simulink model "mcu"  (R2025b)
settings: Solver=FixedStepDiscrete  StartTime=0.0  StopTime=10.0  FixedStep=Ts_inner  RelTol=1e-3
undefined symbols (not defined in the file): controller, imu, mahony, quadcop, safety, Ts_batt, Ts_inner
settings Model: DataDictionary=project.sldd  Creator=Nick  LastModifiedBy=Rakete
settings SolverCC: AutoInsertRateTranBlk=on
settings OptimizationCC: DefaultParameterBehavior=Inlined  EnhancedBackFolding=on  PassReuseOutputArgsAs=Individual arguments  ZeroExternalMemoryAtStartup=off  ZeroInternalMemoryAtStartup=off  OptimizeBlockOrder=speed  DifferentSizesBufferReuse=on  OptimizationCustomize=off  EfficientTunableParamExpr=on
settings DebuggingCC: ParameterTunabilityLossMsg=error
settings HardwareCC: ProdBitPerPointer=32.0  ProdBitPerSizeT=32.0  ProdBitPerPtrDiffT=32.0  ProdLargestAtomicInteger=Long  ProdLargestAtomicFloat=Double  ProdWordSize=32.0  ProdLongLongMode=on  ProdHWDeviceType=ARM Compatible->ARM Cortex-M
settings SFSimCC: MATLABDynamicMemAlloc=off
settings RTWCC: SystemTargetFile=ert.tlc  GenCodeOnly=on  PackageGeneratedCodeAndArtifacts=on  TemplateMakefile=ert_default_tmf  GenerateReport=on  TargetLang=C++  Description=Embedded Coder
settings CodeAppCC: ForceParamTrailComments=on  IgnoreCustomStorageClasses=off  OperatorAnnotations=on  SimulinkDataObjDesc=on  SFDataObjDesc=on  InsertBlockDesc=on
settings ERTTargetCC: RootIOFormat=Structure reference  ERTCustomFileTemplate=example_file_process.tlc  TargetLangStandard=C++11 (ISO)  GenerateSampleERTMain=on  CodeInterfacePackaging=C++ class  SubcomponentCodeInterfacePackaging=C++ class  SupportNonFinite=off

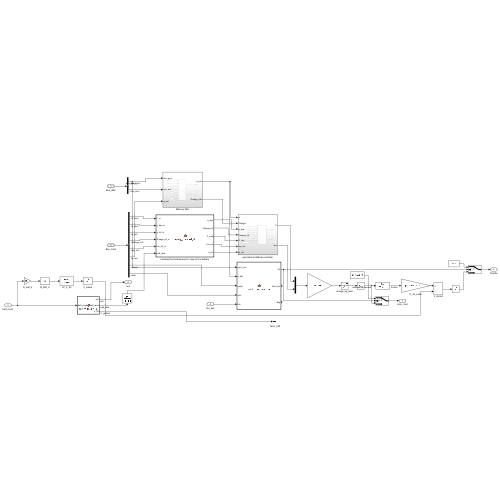
[thumbnail: Simulink's stored preview of the top-level diagram]
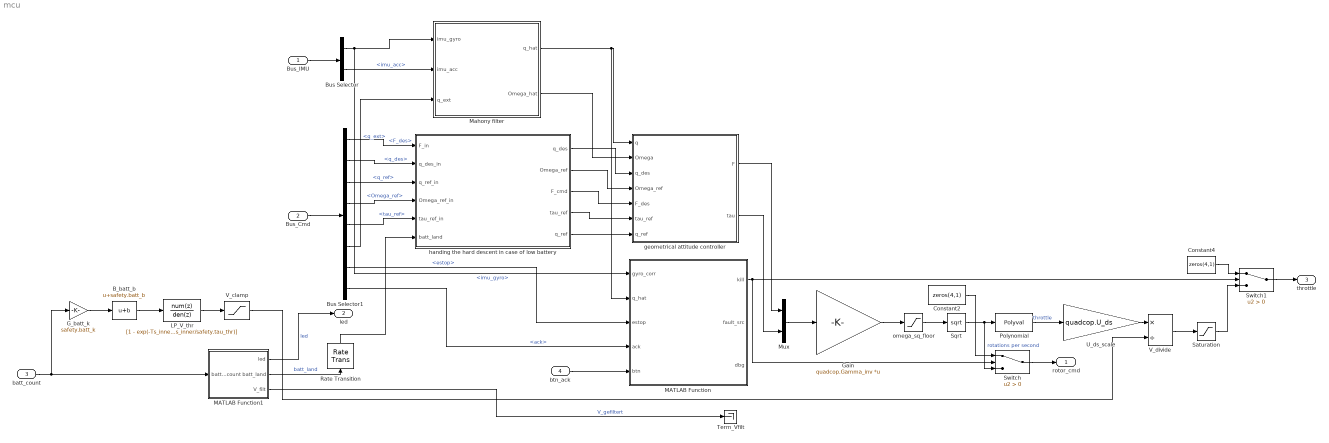
== system mcu ==
  Bus_IMU : Inport  OutDataTypeStr=Bus: Bus_IMU
  Bus_Cmd : Inport  Port=2  OutDataTypeStr=Bus: Bus_Cmd
  batt_count : Inport  Port=3
  btn_ack : Inport  Port=4  OutDataTypeStr=boolean
  B_batt_b : Bias  Bias=safety.batt_b  SaturateOnIntegerOverflow=off
  Bus Selector : BusSelector  OutputSignals=imu_gyro,imu_acc
  Bus Selector1 : BusSelector  OutputSignals=F_des,q_des,q_ref,Omega_ref,tau_ref,q_ext,estop,ack
  Constant2 : Constant  Value=zeros(4,1)
  Constant4 : Constant  Value=zeros(4,1)
  G_batt_k : Gain  Gain=safety.batt_k
  Gain : Gain  Gain=quadcop.Gamma_inv  Multiplication=Matrix(K*u) (u vector)
  LP_V_thr : DiscreteTransferFcn  Numerator=[1 - exp(-Ts_inner/safety.tau_thr)]  Denominator=[1, -exp(-Ts_inner/safety.tau_thr)]  InitialStates=quadcop.V_thr_init  SampleTime=Ts_inner
  MATLAB Function : MATLAB Function  TreatAsAtomicUnit=on
  MATLAB Function1 : MATLAB Function  TreatAsAtomicUnit=on  SystemSampleTime=Ts_batt
  Mahony filter : Subsystem
  Mux : Mux  Inputs=2
  Polynomial : Polyval  Coefs=quadcop.p_from_omega
  Rate Transition : RateTransition  OutPortSampleTime=Ts_inner
  Saturation : Saturate  UpperLimit=100  LowerLimit=0
  Sqrt : Sqrt
  Switch : Switch  Criteria=u2 > Threshold  SaturateOnIntegerOverflow=off  InputSameDT=off
  Switch1 : Switch  Criteria=u2 > Threshold  SaturateOnIntegerOverflow=off  InputSameDT=off
  Term_Vfilt : Terminator
  U_ds_scale : Gain  Gain=quadcop.U_ds
  V_clamp : Saturate  UpperLimit=quadcop.V_thr_max  LowerLimit=quadcop.V_thr_min
  V_divide : Product  Inputs=*/
  geometrical attitude controller : Subsystem
  handing the hard descent in case of low battery : MATLAB Function  TreatAsAtomicUnit=on  SystemSampleTime=Ts_inner
  omega_sq_floor : Saturate  UpperLimit=inf  LowerLimit=0
  rotor_cmd : Outport
  led : Outport  Port=2
  throttle : Outport  Port=3
  wires:
  Bus_IMU/1 -> Bus Selector/1
  geometrical attitude controller/2(tau) -> Mux/2
  Bus Selector/2 -> Mahony filter/2(imu_acc)  "<imu_acc>"
  Bus_Cmd/1 -> Bus Selector1/1
  Bus Selector/1 -> MATLAB Function/1(gyro_corr), Mahony filter/1(imu_gyro)  "<imu_gyro>"
  Bus Selector1/1 -> handing the hard descent in case of low battery/1(F_in)  "<F_des>"
  Bus Selector1/2 -> handing the hard descent in case of low battery/2(q_des_in)  "<q_des>"
  Bus Selector1/3 -> handing the hard descent in case of low battery/3(q_ref_in)  "<q_ref>"
  Bus Selector1/4 -> handing the hard descent in case of low battery/4(Omega_ref_in)  "<Omega_ref>"
  Mux/1 -> Gain/1
  Mahony filter/1(q_hat) -> geometrical attitude controller/1(q), MATLAB Function/2(q_hat)
  Bus Selector1/5 -> handing the hard descent in case of low battery/5(tau_ref_in)  "<tau_ref>"
  handing the hard descent in case of low battery/4(tau_ref) -> geometrical attitude controller/6(tau_ref)
  Bus Selector1/6 -> Mahony filter/3(q_ext)  "<q_ext>"
  Bus Selector1/7 -> MATLAB Function/3(estop)  "<estop>"
  Bus Selector1/8 -> MATLAB Function/4(ack)  "<ack>"
  Rate Transition/1 -> handing the hard descent in case of low battery/6(batt_land)
  Mahony filter/2(Omega_hat) -> geometrical attitude controller/2(Omega)
  Saturation/1 -> Switch1/3
  handing the hard descent in case of low battery/1(q_des) -> geometrical attitude controller/3(q_des)
  handing the hard descent in case of low battery/2(Omega_ref) -> geometrical attitude controller/4(Omega_ref)
  Constant2/1 -> Switch/1
  handing the hard descent in case of low battery/3(F_cmd) -> geometrical attitude controller/5(F_des)
  handing the hard descent in case of low battery/5(q_ref) -> geometrical attitude controller/7(q_ref)
  btn_ack/1 -> MATLAB Function/5(btn)
  geometrical attitude controller/1(F) -> Mux/1
  MATLAB Function/1(kill) -> Switch/2, Switch1/2
  V_divide/1 -> Saturation/1
  Sqrt/1 -> Switch/3, Polynomial/1  "rotations per second"
  Polynomial/1 -> U_ds_scale/1  "throttle"
  Switch/1 -> rotor_cmd/1
  U_ds_scale/1 -> V_divide/1
  Constant4/1 -> Switch1/1
  Switch1/1 -> throttle/1
  Gain/1 -> omega_sq_floor/1
  omega_sq_floor/1 -> Sqrt/1
  MATLAB Function1/3(V_filt) -> Term_Vfilt/1  "V_gefiltert"
  LP_V_thr/1 -> V_clamp/1
  B_batt_b/1 -> LP_V_thr/1
  G_batt_k/1 -> B_batt_b/1
  V_clamp/1 -> V_divide/2
  MATLAB Function1/2(batt_land) -> Rate Transition/1  "batt_land"
  MATLAB Function1/1(led) -> led/1  "led"
  batt_count/1 -> G_batt_k/1, MATLAB Function1/1(batt_count)

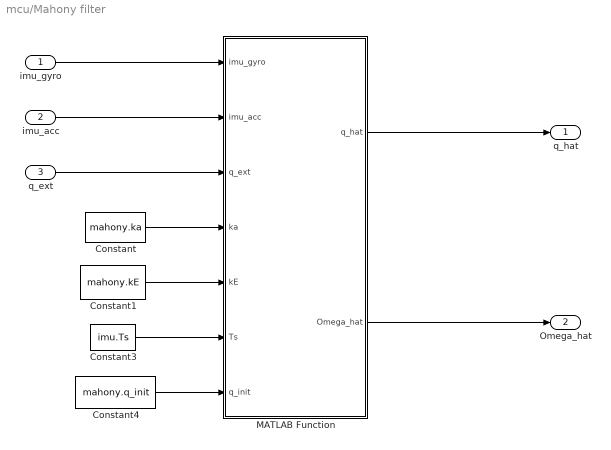
== system mcu/Mahony filter ==
  imu_gyro : Inport
  imu_acc : Inport  Port=2
  q_ext : Inport  Port=3
  Constant : Constant  Value=mahony.ka
  Constant1 : Constant  Value=mahony.kE
  Constant3 : Constant  Value=imu.Ts
  Constant4 : Constant  Value=mahony.q_init
  MATLAB Function : MATLAB Function  TreatAsAtomicUnit=on
  q_hat : Outport
  Omega_hat : Outport  Port=2
  wires:
  MATLAB Function/1(q_hat) -> q_hat/1
  MATLAB Function/2(Omega_hat) -> Omega_hat/1
  imu_gyro/1 -> MATLAB Function/1(imu_gyro)
  imu_acc/1 -> MATLAB Function/2(imu_acc)
  q_ext/1 -> MATLAB Function/3(q_ext)
  Constant/1 -> MATLAB Function/4(ka)
  Constant1/1 -> MATLAB Function/5(kE)
  Constant3/1 -> MATLAB Function/6(Ts)
  Constant4/1 -> MATLAB Function/7(q_init)

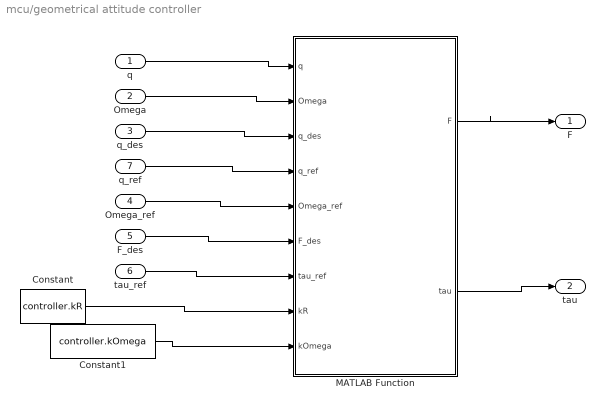
== system mcu/geometrical attitude controller ==
  q : Inport
  Omega : Inport  Port=2
  q_des : Inport  Port=3
  Omega_ref : Inport  Port=4
  F_des : Inport  Port=5
  tau_ref : Inport  Port=6
  q_ref : Inport  Port=7
  Constant : Constant  Value=controller.kR
  Constant1 : Constant  Value=controller.kOmega
  MATLAB Function : MATLAB Function  TreatAsAtomicUnit=on
  F : Outport
  tau : Outport  Port=2
  wires:
  MATLAB Function/1(F) -> F/1
  MATLAB Function/2(tau) -> tau/1
  q/1 -> MATLAB Function/1(q)
  Omega/1 -> MATLAB Function/2(Omega)
  q_des/1 -> MATLAB Function/3(q_des)
  Omega_ref/1 -> MATLAB Function/5(Omega_ref)
  F_des/1 -> MATLAB Function/6(F_des)
  tau_ref/1 -> MATLAB Function/7(tau_ref)
  Constant/1 -> MATLAB Function/8(kR)
  Constant1/1 -> MATLAB Function/9(kOmega)
  q_ref/1 -> MATLAB Function/4(q_ref)

== matlab function mcu/geometrical attitude controller/MATLAB Function ==
  data: q input; F output; Omega input; q_des input; q_ref input; Omega_ref input; F_des input; tau_ref input; kR input; kOmega input; tau output; quadcop parameter
function [F, tau] = geo_attitude_ctrl_sl(q, Omega, q_des, q_ref, Omega_ref, F_des, tau_ref, kR, kOmega, quadcop)
%#codegen
% WRAPPER — code liegt in
% scripts\functions\geo_attitude_ctrl.m - dieser Block ruft sie nur auf
[F, tau] = geo_attitude_ctrl(q, Omega, q_des, q_ref, Omega_ref, F_des, tau_ref, kR, kOmega, quadcop.J);
end

== matlab function mcu/Mahony filter/MATLAB Function ==
  data: imu_gyro input; q_hat output; imu_acc input; q_ext input; ka input; kE input; Ts input; Omega_hat output; q_init input
function [q_hat, Omega_hat] = mahony_filter_sl(imu_gyro, imu_acc, q_ext, ka, kE, Ts, q_init)
%#codegen
% WRAPPER — code liegt in
% scripts\functions\mahony_filter.m - dieser Block ruft sie nur auf
[q_hat, Omega_hat] = mahony_filter(imu_gyro, imu_acc, q_ext, ka, kE, Ts, q_init);
end

== matlab function mcu/MATLAB Function ==
  data: gyro_corr input double size=[3 1]; q_hat input; estop input uint8 size=1; kill output boolean size=1; ack input boolean size=1; btn input; fault_src output uint8 size=1; dbg output size=[3 1]; safety parameter
function [kill, fault_src, dbg] = safety_overspeed_sl(gyro_corr, q_hat, estop, ack, btn, safety)
%#codegen
% WRAPPER  code liegt in
% scripts\functions\safety_overspeed.m - dieser Block ruft sie nur auf
[kill, fault_src, dbg] = safety_overspeed(gyro_corr, q_hat, estop, ack, btn, safety);
end

== matlab function mcu/MATLAB Function1 ==
  data: batt_count input; led output; batt_land output boolean size=[1 1]; V_filt output double size=[1 1]; safety parameter
function [led, batt_land, V_filt] = safety_battery_sl(batt_count, safety)
%#codegen
% WRAPPER — code liegt in
% scripts\functions\safety_battery.m - dieser Block ruft sie nur auf
[led, batt_land, V_filt] = safety_battery(batt_count, safety);
end

== matlab function mcu/handing the hard descent in case of low battery ==
  data: q_des output; Omega_ref output; F_in input; F_cmd output; tau_ref output; q_des_in input; q_ref_in input; Omega_ref_in input; tau_ref_in input; batt_land input; q_ref output; safety parameter
function [q_des, Omega_ref, F_cmd, tau_ref, q_ref] = safety_landcmd_sl(F_in, q_des_in, q_ref_in, Omega_ref_in, tau_ref_in, batt_land, safety)
%#codegen
% WRAPPER — code liegt in
% scripts\functions\safety_landcmd.m - dieser Block ruft sie nur auf
[q_des, Omega_ref, F_cmd, tau_ref, q_ref] = safety_landcmd(F_in, q_des_in, q_ref_in, Omega_ref_in, tau_ref_in, batt_land, safety);
end
